simulink model "KF_Pendulum"  (R2016b)
settings: Solver=FixedStepAuto  StartTime=0.0  StopTime=15  FixedStep=0.01  RelTol=1e-3
values from neighbouring files (symbols this model uses):
  A = [0 1; -g/l 0]    [Pendulum.m]    (also in Pendulum_Noise.m = [0 1;-1 0])
  B = [0; tau/(m*l^2)]    [Pendulum.m]    (also in Pendulum_Noise.m = [0; 1])
  C = [1 0]    [Pendulum.m]    (also in Pendulum_Noise.m = [0 1])
  D = 0    [Pendulum.m]    (also in Pendulum_Noise.m)
  g = 9.81    [Pendulum.m]    (also in Pendulum_Noise.m)
  l = 1    [Pendulum.m]    (also in Pendulum_Noise.m)
  m = 1    [Pendulum.m]    (also in Pendulum_Noise.m)
  tau = 1    [Pendulum.m]    (also in Pendulum_Noise.m)
  x0 = [1 1]    [Pendulum.m]
undefined symbols (not defined in the file or in its folder): Continuous, Time
libraries: simulink x2, ctrlSharedLib x1
settings Model: Creator=Daniel  LastModifiedBy=Daniel

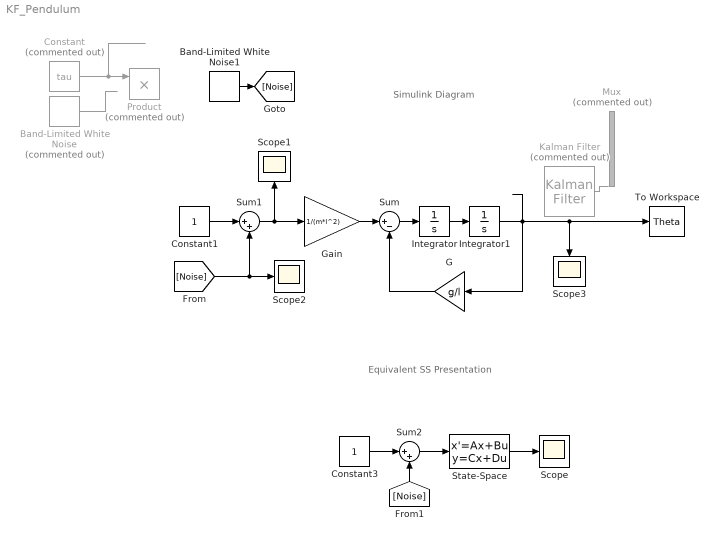
== system KF_Pendulum ==
  note: Equivalent SS Presentation
  note: Simulink Diagram
  Band-Limited White Noise : simulink/Sources/Band-Limited White Noise  Commented=on  Cov=[0.01]  Ts=0.01  seed=[23341]
  Band-Limited White Noise1 : simulink/Sources/Band-Limited White Noise  Cov=0.01  Ts=0.01  seed=[23341]
  Constant : Constant  Commented=on  Value=tau
  Constant1 : Constant
  Constant3 : Constant
  G : Gain  Gain=g/l
  Gain : Gain  Gain=1/(m*l^2)
  Integrator : Integrator
  Integrator1 : Integrator
  Kalman Filter : ctrlSharedLib/Kalman Filter  Commented=on  TimeDomain=Continuous-Time  UseCurrentEstimator=on  ModelSource=Individual A, B, C, D matrices  ModelSourceVariable=ss(0.95,1,1,0,1)  A=A  B=B  C=C  D=D  NumberOfStates=1  NumberOfInputs=1  NumberOfOutputs=1  InitialEstimateSource=Input port  X0=x0  P0=10  UseK=off  UseGH=off  NumberOfProcessNoiseInputs=1  G=1  TimeInvariantG=on  H=0  TimeInvariantH=on  Q=0.05  TimeInvariantQ=on  R=1  TimeInvariantR=on  N=0  TimeInvariantN=on  AddInputPort=on  AddEnablePort=off  ExternalReset=none  OutputEstimatedY=off  OutputP=off  Ts=-1
  Mux : Mux  Commented=on  Inputs=2
  Product : Product  Commented=on
  Scope{,1..3} (4 alike) : Scope
  State-Space : StateSpace  A=A  B=B  C=C  D=D  X0=x0
  Sum : Sum  Inputs=|+-
  Sum1 : Sum  Inputs=|++
  Sum2 : Sum  Inputs=|++
  To Workspace : ToWorkspace  VariableName=Theta  SaveFormat=Timeseries  SampleTime=-1
  wires:
  Gain/1 -> Sum/1
  Integrator/1 -> Integrator1/1
  Sum/1 -> Integrator/1
  G/1 -> Sum/2
  Band-Limited White Noise/1 -> ?
  Constant/1 -> Product/1
  Kalman Filter/1 -> ?
  Integrator1/1 -> Scope3/1, To Workspace/1, G/1
  Constant1/1 -> Sum1/1
  Sum2/1 -> State-Space/1
  State-Space/1 -> Scope/1
  Sum1/1 -> Scope1/1, Gain/1
  Constant3/1 -> Sum2/1
  [Noise] -> Sum1/2, Scope2/1
  Band-Limited White Noise1/1 -> [Noise]
  [Noise] -> Sum2/2
